simulink model "adc_test"  (Simulink 7.0)
settings: Solver=ode45  StartTime=0.0  StopTime=100  RelTol=1e-3
libraries: xbsIndex_r4 x8, xps_library x4, dspsigops x2, isi_correlator_lib x2
settings Model: Creator=wjm  LastModifiedBy=wjm

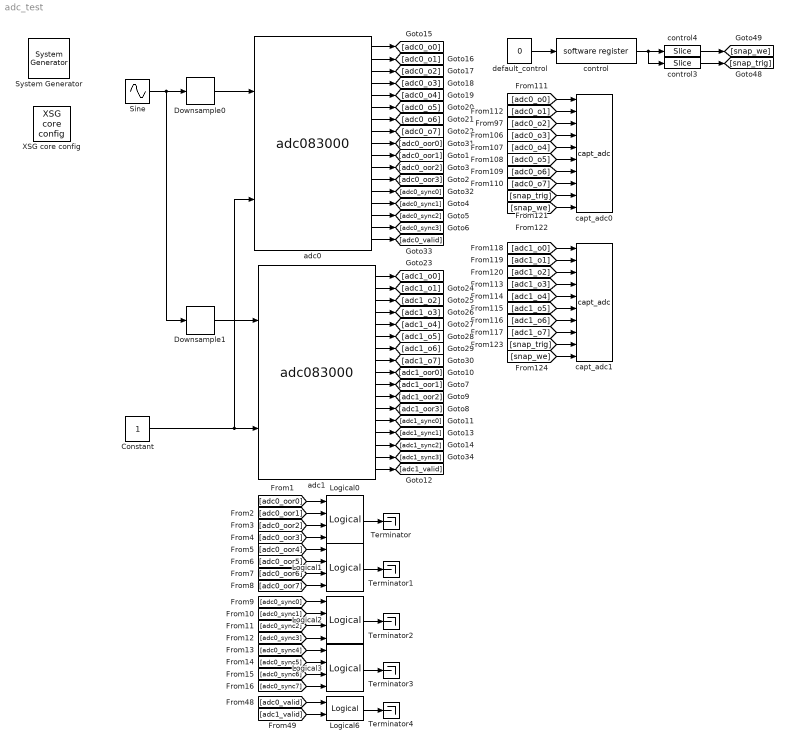
== system adc_test ==
  " System Generator" : xbsIndex_r4/ System Generator  Tag=genX  SystemSampleTime=-1  xilinxfamily=virtex5  part=xc5vsx95t  speed=-1  package=ff1136  synthesis_tool=XST  clock_wrapper=Clock Enables  directory=./netlist  testbench=off  simulink_period=1  sysclk_period=100  dcm_input_clock_period=100  incr_netlist=off  trim_vbits=Everywhere in SubSystem  dbl_ovrd=According to Block Masks  core_generation=According to Block Masks  run_coregen=off  deprecated_control=off  eval_field=0  block_type=sysgen
      settings: block_version=10.1.3
  Constant : Constant  OutDataType=sfix(16)  OutScaling=2^0  SampleTime=1
  Downsample0 : dspsigops/Downsample  N=2  phase=1  ic=0  smode=Allow multirate  fmode=Maintain input frame size
  Downsample1 : dspsigops/Downsample  N=2  phase=0  ic=0  smode=Allow multirate  fmode=Maintain input frame size
  Logical{0..3} (4 alike) : xbsIndex_r4/Logical  logical_function=OR  inputs=4  en=off  latency=1  precision=Full  arith_type=Unsigned  n_bits=8  bin_pt=2  align_bp=on  dbl_ovrd=off  block_type=logical
      settings: xl_area=[0, 0, 0, 0, 0, 0, 0]
  Logical6 : xbsIndex_r4/Logical  logical_function=AND  inputs=2  en=off  latency=0  precision=Full  arith_type=Unsigned  n_bits=1  bin_pt=0  align_bp=on  dbl_ovrd=off  block_type=logical
      settings: block_version=10.1.1
  Sine : Sin  Amplitude=.9  Frequency=100*(2*pi/375)  SampleTime=1/16
  Terminator{,1..4} (5 alike) : Terminator
  XSG core config : xps_library/XSG core config  Tag=xps:xsg  SystemSampleTime=-1  hw_sys=ROACH:sx95t  ibob_linux=off  clk_src=adc0_clk  iBOB_clk_src=sys_clk  BEE2_ctrl_clk_src=sys_clk  BEE2_usr_clk_src=sys_clk  ROACH_clk_src=adc0_clk  CORR_clk_src=sys_clk  gpio_clk_io_group=iBOB:sma  gpio_clk_bit_index=0  clk_rate=200  sample_period=1  synthesis_tool=XST  mpc_type=powerpc440_ext
  adc0 : xps_library/adc083000  Tag=xps:adc083000  SystemSampleTime=-1  adc_brd=adc0  adc_clk_rate=800  adc_interleave=on  sample_period=1
  adc1 : xps_library/adc083000  Tag=xps:adc083000  SystemSampleTime=-1  adc_brd=adc1  adc_clk_rate=800  adc_interleave=on  sample_period=1
  capt_adc0 : isi_correlator_lib/capt_adc  SystemSampleTime=-1
  capt_adc1 : isi_correlator_lib/capt_adc  SystemSampleTime=-1
  control : xps_library/software register  Tag=xps:sw_reg  SystemSampleTime=-1  io_dir=From Processor  arith_type=Unsigned  bitwidth=32  bin_pt=0  sample_period=1  gw_name=adc_test_control_user_data_out
      link override corr_3ghz_10_1_corr_id_user_data_out: arith_type=Unsigned  n_bits=32  bin_pt=0  period=1
      link override corr_3ghz_10_1_exp_corr_id_user_data_out: arith_type=Unsigned  n_bits=32  bin_pt=0  period=1
      link override isi_corr_eq_coeff_user_data_out: arith_type=Unsigned  n_bits=32  bin_pt=0  period=1
      link override isi_correlator_control_user_data_out: arith_type=Unsigned  n_bits=32  bin_pt=0  period=1
      link override isi_correlator_cropped_control_user_data_out: arith_type=Unsigned  n_bits=32  bin_pt=0  period=1
      link override isi_correlator_eq_coeff_user_data_out: arith_type=Unsigned  n_bits=32  bin_pt=0  period=1
  control3 : xbsIndex_r4/Slice  nbits=1  boolean_output=on  mode=Lower Bit Location + Width  bit1=0  base1=MSB of Input  bit0=3  base0=LSB of Input  dbl_ovrd=off  block_type=slice
      settings: infoedit="Extracts a given range of bits from each input sample and presents it at the output.  The output type is ordinarily unsigned with binary point at zero, but can be Boolean when the slice is one bit wide.<P><P>Hardware notes: In hardware this block costs nothing."  block_version=10.1.3
  control4 : xbsIndex_r4/Slice  nbits=1  boolean_output=on  mode=Lower Bit Location + Width  bit1=0  base1=MSB of Input  bit0=4  base0=LSB of Input  dbl_ovrd=off  block_type=slice
      settings: infoedit="Extracts a given range of bits from each input sample and presents it at the output.  The output type is ordinarily unsigned with binary point at zero, but can be Boolean when the slice is one bit wide.<P><P>Hardware notes: In hardware this block costs nothing."  block_version=10.1.3
  default_control : Constant  Value=0  OutDataType=sfix(16)  OutScaling=2^0  SampleTime=1
  wires:
  adc0/1 -> [adc0_o0]
  adc0/2 -> [adc0_o1]
  adc0/3 -> [adc0_o2]
  adc0/4 -> [adc0_o3]
  adc0/5 -> [adc0_o4]
  adc0/6 -> [adc0_o5]
  adc0/7 -> [adc0_o6]
  adc0/8 -> [adc0_o7]
  adc0/9 -> [adc0_oor0]
  adc0/10 -> [adc0_oor1]
  adc0/11 -> [adc0_oor2]
  adc0/12 -> [adc0_oor3]
  adc0/13 -> [adc0_sync0]
  adc0/14 -> [adc0_sync1]
  adc0/15 -> [adc0_sync2]
  adc0/16 -> [adc0_sync3]
  adc0/17 -> [adc0_valid]
  adc1/1 -> [adc1_o0]
  adc1/2 -> [adc1_o1]
  adc1/3 -> [adc1_o2]
  adc1/4 -> [adc1_o3]
  adc1/5 -> [adc1_o4]
  adc1/6 -> [adc1_o5]
  adc1/7 -> [adc1_o6]
  adc1/8 -> [adc1_o7]
  adc1/9 -> [adc1_oor0]
  adc1/10 -> [adc1_oor1]
  adc1/11 -> [adc1_oor2]
  adc1/12 -> [adc1_oor3]
  adc1/13 -> [adc1_sync0]
  adc1/14 -> [adc1_sync1]
  adc1/15 -> [adc1_sync2]
  adc1/16 -> [adc1_sync3]
  adc1/17 -> [adc1_valid]
  Downsample0/1 -> adc0/1
  Downsample1/1 -> adc1/1
  Sine/1 -> Downsample0/1, Downsample1/1
  Constant/1 -> adc1/2, adc0/2
  [adc0_oor0] -> Logical0/1
  [adc0_oor1] -> Logical0/2
  [adc0_oor2] -> Logical0/3
  [adc0_oor3] -> Logical0/4
  [adc0_oor4] -> Logical1/1
  [adc0_oor5] -> Logical1/2
  [adc0_oor6] -> Logical1/3
  [adc0_oor7] -> Logical1/4
  [adc0_sync0] -> Logical2/1
  [adc0_sync1] -> Logical2/2
  [adc0_sync2] -> Logical2/3
  [adc0_sync3] -> Logical2/4
  [adc0_sync4] -> Logical3/1
  [adc0_sync5] -> Logical3/2
  [adc0_sync6] -> Logical3/3
  [adc0_sync7] -> Logical3/4
  Logical0/1 -> Terminator/1
  Logical1/1 -> Terminator1/1
  Logical2/1 -> Terminator2/1
  Logical3/1 -> Terminator3/1
  [adc0_valid] -> Logical6/1
  [adc1_valid] -> Logical6/2
  Logical6/1 -> Terminator4/1
  default_control/1 -> control/1
  control/1 -> control4/1, control3/1
  [adc0_o0] -> capt_adc0/1
  [adc0_o1] -> capt_adc0/2
  [adc0_o2] -> capt_adc0/3
  [adc0_o3] -> capt_adc0/4
  [adc0_o4] -> capt_adc0/5
  [adc0_o5] -> capt_adc0/6
  [adc0_o6] -> capt_adc0/7
  [adc0_o7] -> capt_adc0/8
  [adc1_o0] -> capt_adc1/1
  [adc1_o1] -> capt_adc1/2
  [adc1_o2] -> capt_adc1/3
  [adc1_o3] -> capt_adc1/4
  [adc1_o4] -> capt_adc1/5
  [adc1_o5] -> capt_adc1/6
  [adc1_o6] -> capt_adc1/7
  [adc1_o7] -> capt_adc1/8
  [snap_trig] -> capt_adc0/9
  [snap_we] -> capt_adc0/10
  [snap_trig] -> capt_adc1/9
  [snap_we] -> capt_adc1/10
  control4/1 -> [snap_we]
  control3/1 -> [snap_trig]
